simulink model "BLDCspeedcontrollerForGeneralLC"  (R2018b)
settings: Solver=ode15s  StartTime=0  StopTime=10  MaxStep=0.0001  MinStep=1e-9  RelTol=1e-6  AbsTol=1e-9
values from neighbouring files (symbols this model uses):
  battery =     [battery.mat]
  brake =     [brake.mat]
  PE =     [PE.mat]
  pmsm =     [bldc.mat]
undefined symbols (not defined in the file or in its folder): Controller, mech, sigbuilder_block
libraries: simulink x3, simulink_extras x1
settings Model: SimulationMode=accelerator  Creator=dimitriosvogiatzis  LastModifiedBy=dimitriosvogiatzis
settings SolverCC: AutoScaleAbsTol=off  InitialStep=1e-8  MaxConsecutiveZCs=100  MaxConsecutiveMinStep=100  ZeroCrossAlgorithm=Adaptive  AlgebraicLoopSolver=LineSearch
settings DebuggingCC: IgnoredZcDiagnostic=none
settings CodeAppCC: StateflowObjectComments=on

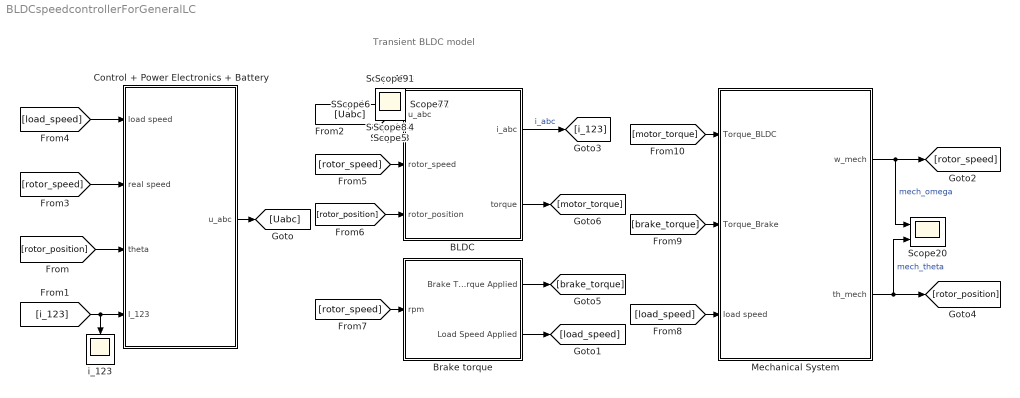
== system BLDCspeedcontrollerForGeneralLC ==
  note: Transient BLDC model
  BLDC : Subsystem
  Brake torque : Subsystem
  Control + Power Electronics + Battery : Subsystem
  Mechanical System : Subsystem
  Scope20 : Scope  NumInputPorts=2
  i_123 : Scope
  Scope{,1..19,21..47} (47 alike) : Scope
  wires:
  BLDC/1(i_abc) -> [i_123]  "i_abc"
  Mechanical System/1(w_mech) -> Scope20/1, [rotor_speed]  "mech_omega"
  Brake torque/1(Brake Torque Applied) -> [brake_torque]
  Mechanical System/2(th_mech) -> Scope20/2, [rotor_position]  "mech_theta"
  [load_speed] -> Control + Power Electronics + Battery/1(load speed)
  [rotor_speed] -> Control + Power Electronics + Battery/2(real speed)
  [rotor_position] -> Control + Power Electronics + Battery/3(theta)
  [i_123] -> Control + Power Electronics + Battery/4(I_123), i_123/1
  [rotor_speed] -> BLDC/2(rotor_speed)
  BLDC/2(torque) -> [motor_torque]
  [rotor_position] -> BLDC/3(rotor_position)
  [rotor_speed] -> Brake torque/1(rpm)
  Brake torque/2(Load Speed Applied) -> [load_speed]
  Control + Power Electronics + Battery/1(u_abc) -> [Uabc]
  [Uabc] -> BLDC/1(u_abc)
  [load_speed] -> Mechanical System/3(load speed)
  [brake_torque] -> Mechanical System/2(Torque_Brake)
  [motor_torque] -> Mechanical System/1(Torque_BLDC)

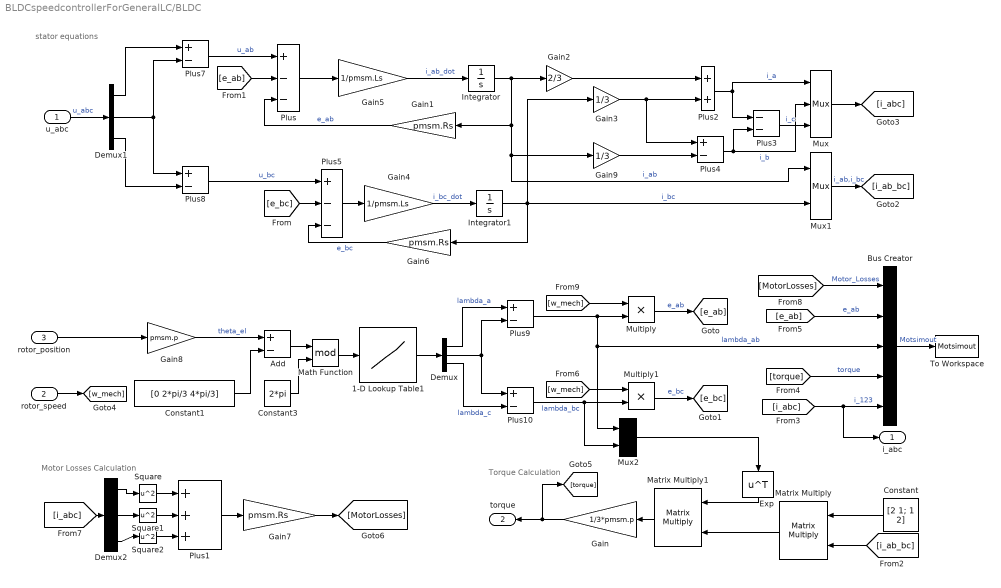
== system BLDCspeedcontrollerForGeneralLC/BLDC ==
  note: Motor Losses Calculation
  note: stator equations
  note: Torque Calculation
  u_abc : Inport
  rotor_speed : Inport  Port=2
  rotor_position : Inport  Port=3
  1-D Lookup Table1 : Lookup_n-D  NumberOfTableDimensions=1  BreakpointsForDimension1=pmsm.phi_tab  Table=pmsm.dlambda_tab  InternalRulePriority=Speed  RndMeth=Simplest  InputSameDT=on
  Add : Sum  Inputs=+-
  Bus Creator : BusCreator  Inputs=5
  Constant : Constant  Value=[2 1; 1 2]
  Constant1 : Constant  Value=[0 2*pi/3 4*pi/3]
  Constant3 : Constant  Value=2*pi
  Demux : Demux  Outputs=3
  Demux1 : Demux  Outputs=3
  Demux2 : Demux  Outputs=3
  Exp : Math  Operator=transpose  OutputSignalType=real  SaturateOnIntegerOverflow=on
  Gain : Gain  Gain=1/3*pmsm.p
  Gain1 : Gain  Gain=pmsm.Rs
  Gain2 : Gain  Gain=2/3
  Gain3 : Gain  Gain=1/3
  Gain4 : Gain  Gain=1/pmsm.Ls
  Gain5 : Gain  Gain=1/pmsm.Ls
  Gain6 : Gain  Gain=pmsm.Rs
  Gain7 : Gain  Gain=pmsm.Rs
  Gain8 : Gain  Gain=pmsm.p
  Gain9 : Gain  Gain=1/3
  Integrator : Integrator
  Integrator1 : Integrator
  Math Function : Math  Operator=mod  SaturateOnIntegerOverflow=on
  Matrix Multiply : Product  Multiplication=Matrix(*)
  Matrix Multiply1 : Product  Multiplication=Matrix(*)
  Multiply : Product
  Multiply1 : Product
  Mux : Mux  Inputs=3
  Mux1 : Mux  Inputs=2
  Mux2 : Mux  Inputs=2
  Plus : Sum  Inputs=+--
  Plus1 : Sum  Inputs=+++
  Plus{4,7..10} (5 alike) : Sum  Inputs=+-
  Plus2 : Sum
  Plus3 : Sum  Inputs=--
  Plus5 : Sum  Inputs=+--
  Square : Math  Operator=square  SaturateOnIntegerOverflow=on
  Square1 : Math  Operator=square  SaturateOnIntegerOverflow=on
  Square2 : Math  Operator=square  SaturateOnIntegerOverflow=on
  To Workspace : ToWorkspace  VariableName=Motsimout  SaveFormat=Timeseries  SampleTime=-1
  i_abc : Outport
  torque : Outport  Port=2
  wires:
  Multiply/1 -> [e_ab]  "e_ab"
  Matrix Multiply/1 -> Matrix Multiply1/2
  Mux2/1 -> Exp/1
  Demux/2 -> Plus9/2, Plus10/1
  Plus10/1 -> Multiply1/2, Mux2/2  "lambda_bc"
  Constant/1 -> Matrix Multiply/1
  [e_bc] -> Plus5/2
  Gain6/1 -> Plus5/3  "e_bc"
  Plus4/1 -> Mux/2, Plus3/2  "i_b"
  1-D Lookup Table1/1 -> Demux/1
  [i_ab_bc] -> Matrix Multiply/2
  Matrix Multiply1/1 -> Gain/1
  Mux1/1 -> [i_ab_bc]  "i_ab,i_bc"
  [e_ab] -> Plus/2
  [i_abc] -> i_abc/1, Bus Creator/5  "i_123"
  Add/1 -> Math Function/1
  Exp/1 -> Matrix Multiply1/1
  Demux/3 -> Plus10/2  "lambda_c"
  [w_mech] -> Multiply/1
  Constant1/1 -> Add/2
  Demux/1 -> Plus9/1  "lambda_a"
  Gain8/1 -> Add/1  "theta_el"
  Math Function/1 -> 1-D Lookup Table1/1
  Gain3/1 -> Plus4/1, Plus2/2
  Plus2/1 -> Mux/1, Plus3/1  "i_a"
  Gain9/1 -> Plus4/2
  Integrator/1 -> Mux1/1, Gain9/1, Gain1/1, Gain2/1  "i_ab"
  Gain1/1 -> Plus/3  "e_ab"
  Gain2/1 -> Plus2/1
  Gain5/1 -> Integrator/1  "i_ab_dot"
  rotor_speed/1 -> [w_mech]
  Gain4/1 -> Integrator1/1  "i_bc_dot"
  Multiply1/1 -> [e_bc]  "e_bc"
  [w_mech] -> Multiply1/1
  Integrator1/1 -> Gain6/1, Mux1/2, Gain3/1  "i_bc"
  Plus/1 -> Gain5/1
  Mux/1 -> [i_abc]
  Plus9/1 -> Mux2/1, Bus Creator/3, Multiply/2  "lambda_ab"
  Plus5/1 -> Gain4/1
  Constant3/1 -> Math Function/2
  Demux1/3 -> Plus8/2
  Demux1/1 -> Plus7/1
  Plus8/1 -> Plus5/1  "u_bc"
  Demux1/2 -> Plus8/1, Plus7/2
  Plus7/1 -> Plus/1  "u_ab"
  u_abc/1 -> Demux1/1  "u_abc"
  rotor_position/1 -> Gain8/1
  Bus Creator/1 -> To Workspace/1  "Motsimout"
  Plus3/1 -> Mux/3  "i_c"
  Gain/1 -> [torque], torque/1
  [torque] -> Bus Creator/4  "torque"
  [e_ab] -> Bus Creator/2  "e_ab"
  [i_abc] -> Demux2/1
  Demux2/1 -> Square/1
  Plus1/1 -> Gain7/1
  Gain7/1 -> [MotorLosses]
  [MotorLosses] -> Bus Creator/1  "Motor_Losses"
  Square/1 -> Plus1/1
  Demux2/2 -> Square1/1
  Square1/1 -> Plus1/2
  Square2/1 -> Plus1/3
  Demux2/3 -> Square2/1

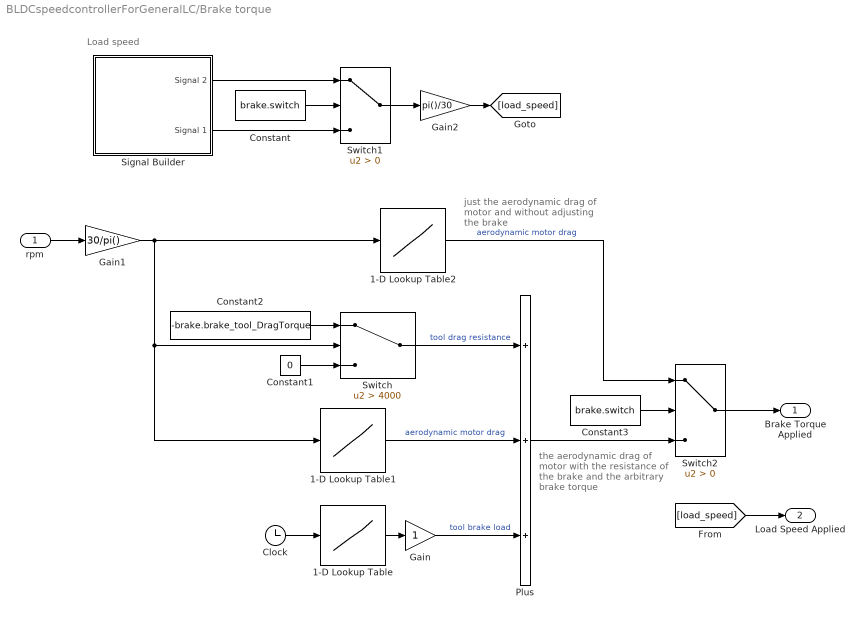
== system BLDCspeedcontrollerForGeneralLC/Brake torque ==
  note: the aerodynamic drag of motor with the resistance of the brake and the arbitrary brake torque
  note: just the aerodynamic drag of motor and without adjusting the brake
  note: Load speed
  rpm : Inport
  1-D Lookup Table : Lookup_n-D  NumberOfTableDimensions=1  BreakpointsForDimension1=brake.brake_time_small  Table=-brake.brake_torque_small  InternalRulePriority=Speed  RndMeth=Simplest  InputSameDT=on
  1-D Lookup Table1 : Lookup_n-D  NumberOfTableDimensions=1  BreakpointsForDimension1=[0,5000,7000,9000,10000,11500,12000]  Table=-1.6*[0,0.28,0.37,0.45,0.5,0.58,0.68]  InternalRulePriority=Speed  RndMeth=Simplest  InputSameDT=on
  1-D Lookup Table2 : Lookup_n-D  NumberOfTableDimensions=1  BreakpointsForDimension1=[0,5000,7000,9000,10000,11500,13000]  Table=-1.6*[0,0.28,0.37,0.45,0.5,0.58,0.68]  InternalRulePriority=Speed  RndMeth=Simplest  InputSameDT=on
  Clock : Clock
  Constant : Constant  Value=brake.switch
  Constant1 : Constant  Value=0
  Constant2 : Constant  Value=-brake.brake_tool_DragTorque
  Constant3 : Constant  Value=brake.switch
  Gain : Gain
  Gain1 : Gain  Gain=30/pi()
  Gain2 : Gain  Gain=pi()/30
  Plus : Sum  Inputs=+++
  Signal Builder : Subsystem  Tag=STV Subsys  LoadFcn=sigbuilder_block('load');  StartFcn=sigbuilder_block('start');  StopFcn=sigbuilder_block('stop');  ClipboardFcn=sigbuilder_block('clipboard');  mask(Sigbuilder block){tuvar=[0:10]}
      mask help: Simulink:masks:SigbuilderBlock_MD
      mask init:
      | if ~strcmp(get_param(bdroot(gcbh),'SimulationStatus'),'stopped') tuvar = sigbuilder_block('maskInit'); end
      settings: CopyFcn=sigbuilder_block('copy');  DeleteFcn=sigbuilder_block('delete');  ModelCloseFcn=sigbuilder_block('modelClose');  PreSaveFcn=sigbuilder_block('preSave');  PauseFcn=sigbuilder_block('pause');  ContinueFcn=sigbuilder_block('continue');  NameChangeFcn=sigbuilder_block('namechange');  OpenFcn=sigbuilder_block('open',[6 30 1428 681.75 ]);  CloseFcn=sigbuilder_block('close');
      mask Display: plot(0, 0, 100, 100,[2, 2, 32, 32, 2], [68, 8, 8, 68, 68],[32, 2], [38, 38], [32, 19, 2],[53, 60, 44], [32, 17, 17, 2],[16, 16, 31, 31]);txt = getActiveGroup(gcbh);text(2, 100, txt,'verticalAlignment', 'top');
  Switch : Switch  Criteria=u2 > Threshold  Threshold=4000
  Switch1 : Switch  Criteria=u2 > Threshold
  Switch2 : Switch  Criteria=u2 > Threshold
  Brake Torque Applied : Outport
  Load Speed Applied : Outport  Port=2
  wires:
  1-D Lookup Table/1 -> Gain/1
  1-D Lookup Table2/1 -> Switch2/1  "aerodynamic motor drag"
  Gain/1 -> Plus/3  "tool brake load"
  Switch2/1 -> Brake Torque Applied/1
  Clock/1 -> 1-D Lookup Table/1
  Plus/1 -> Switch2/3
  1-D Lookup Table1/1 -> Plus/2  "aerodynamic motor drag"
  rpm/1 -> Gain1/1
  Gain1/1 -> 1-D Lookup Table2/1, 1-D Lookup Table1/1, Switch/2
  Constant1/1 -> Switch/3
  Constant2/1 -> Switch/1
  Switch/1 -> Plus/1  "tool drag resistance"
  Signal Builder/2(Signal 1) -> Switch1/3
  Gain2/1 -> [load_speed]
  Switch1/1 -> Gain2/1
  Signal Builder/1(Signal 2) -> Switch1/1
  [load_speed] -> Load Speed Applied/1
  Constant/1 -> Switch1/2
  Constant3/1 -> Switch2/2

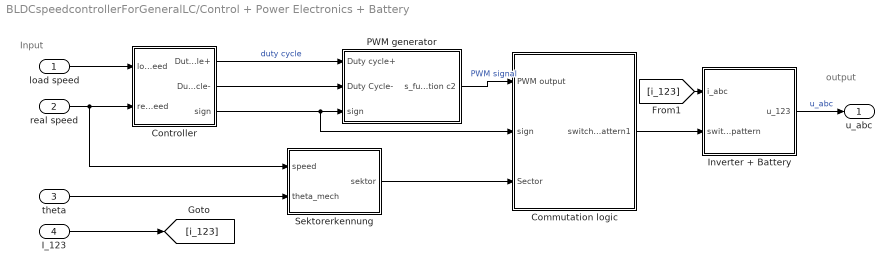
== system BLDCspeedcontrollerForGeneralLC/Control + Power Electronics + Battery ==
  note: output
  note: Input
  load speed : Inport
  real speed : Inport  Port=2
  theta : Inport  Port=3
  I_123 : Inport  Port=4
  Commutation logic : Subsystem
  Controller : Subsystem
  Inverter + Battery : Subsystem
  PWM generator : Subsystem
  Sektorerkennung : Subsystem
  u_abc : Outport
  wires:
  load speed/1 -> Controller/1(load speed)
  theta/1 -> Sektorerkennung/2(theta_mech)
  [i_123] -> Inverter + Battery/1(i_abc)
  Sektorerkennung/1(sektor) -> Commutation logic/3(Sector)
  Controller/1(Duty Cycle+) -> PWM generator/1(Duty cycle+)  "duty cycle"
  Commutation logic/1(switching pattern1) -> Inverter + Battery/2(switching pattern)
  Inverter + Battery/1(u_123) -> u_abc/1  "u_abc"
  real speed/1 -> Sektorerkennung/1(speed), Controller/2(real speed)
  Controller/3(sign) -> Commutation logic/2(sign), PWM generator/3(sign)
  PWM generator/1(s_function c2) -> Commutation logic/1(PWM output)  "PWM signal"
  Controller/2(Duty Cycle-) -> PWM generator/2(Duty Cycle-)
  I_123/1 -> [i_123]

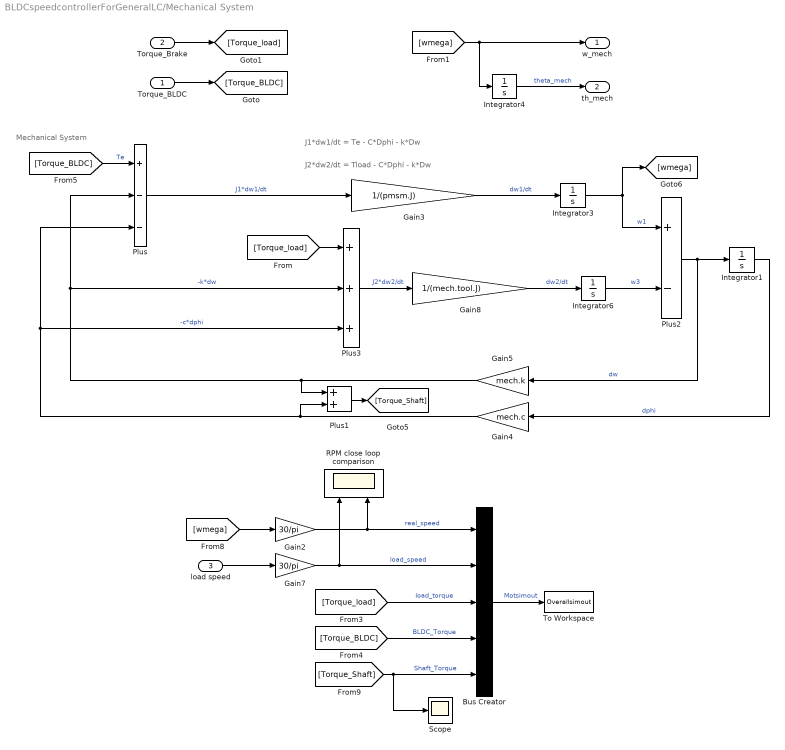
== system BLDCspeedcontrollerForGeneralLC/Mechanical System ==
  note: Mechanical System
  note: J1*dw1/dt = Te - C*Dphi - k*Dw
  note: J2*dw2/dt = Tload - C*Dphi - k*Dw
  Torque_BLDC : Inport
  Torque_Brake : Inport  Port=2
  load speed : Inport  Port=3
  Bus Creator : BusCreator  Inputs=5
  Gain2 : Gain  Gain=30/pi
  Gain3 : Gain  Gain=1/(pmsm.J)
  Gain4 : Gain  Gain=mech.c
  Gain5 : Gain  Gain=mech.k
  Gain7 : Gain  Gain=30/pi
  Gain8 : Gain  Gain=1/(mech.tool.J)
  Integrator{1,3..4,6} (4 alike) : Integrator
  Plus : Sum  Inputs=+--
  Plus1 : Sum
  Plus2 : Sum  Inputs=+-
  Plus3 : Sum  Inputs=+++
  RPM close loop comparison : Scope  NumInputPorts=2
  Scope : Scope
  To Workspace : ToWorkspace  VariableName=Overallsimout  SaveFormat=Timeseries  SampleTime=-1
  w_mech : Outport
  th_mech : Outport  Port=2
  wires:
  Torque_Brake/1 -> [Torque_load]
  Torque_BLDC/1 -> [Torque_BLDC]
  Integrator4/1 -> th_mech/1  "theta_mech"
  Gain4/1 -> Plus1/2, Plus3/3, Plus/3  "-c*dphi"
  Integrator1/1 -> Gain4/1  "dphi"
  Plus1/1 -> [Torque_Shaft]
  Plus2/1 -> Integrator1/1, Gain5/1  "dw"
  Gain3/1 -> Integrator3/1  "dw1/dt"
  Plus/1 -> Gain3/1  "J1*dw1/dt"
  [Torque_BLDC] -> Plus/1  "Te"
  Integrator3/1 -> [wmega], Plus2/1  "w1"
  Gain5/1 -> Plus1/1, Plus3/2, Plus/2  "-k*dw"
  Gain7/1 -> RPM close loop comparison/1, Bus Creator/2  "load_speed"
  Bus Creator/1 -> To Workspace/1  "Motsimout"
  [Torque_load] -> Bus Creator/3  "load_torque"
  [wmega] -> Gain2/1
  load speed/1 -> Gain7/1
  Gain2/1 -> RPM close loop comparison/2, Bus Creator/1  "real_speed"
  [Torque_BLDC] -> Bus Creator/4  "BLDC_Torque"
  [Torque_Shaft] -> Scope/1, Bus Creator/5  "Shaft_Torque"
  [Torque_load] -> Plus3/1
  Plus3/1 -> Gain8/1  "J2*dw2/dt"
  Gain8/1 -> Integrator6/1  "dw2/dt"
  Integrator6/1 -> Plus2/2  "w3"
  [wmega] -> w_mech/1, Integrator4/1

== system BLDCspeedcontrollerForGeneralLC/Brake torque/Signal Builder ==
  Demux : Demux  Tag=STV Demux  Outputs=2
  FromWs : FromWorkspace  Tag=STV FromWs  VariableName=tuvar  SampleTime=0
      SigBuilderData=|
      | common.afterFinalStr = 'Extrapolate'
      | common.sampleTime = 0
      | dataSet.timeRange = [0 10]
      | dataSet.name = 'Group 1'
      | sbobj.Groups.Name = 'Group 1'
      | sbobj.Groups.Signals(1).Name = 'Signal 2'
      | sbobj.Groups.Signals(1).XData = [0 10]
      | sbobj.Groups.Signals(1).YData = [0 200000]
      | sbobj.Groups.Signals(2).Name = 'Signal 1'
      | sbobj.Groups.Signals(2).XData = [0 1.5 3 3.5 5 5.5 8 9 10]
      | sbobj.Groups.Signals(2).YData = [0 4000 4000 6000 6000 8000 8050 10000 0]
  Signal 2 : Outport  Tag=STV Outport
  Signal 1 : Outport  Tag=STV Outport  Port=2
  wires:
  FromWs/1 -> Demux/1
  Demux/1 -> Signal 2/1
  Demux/2 -> Signal 1/1

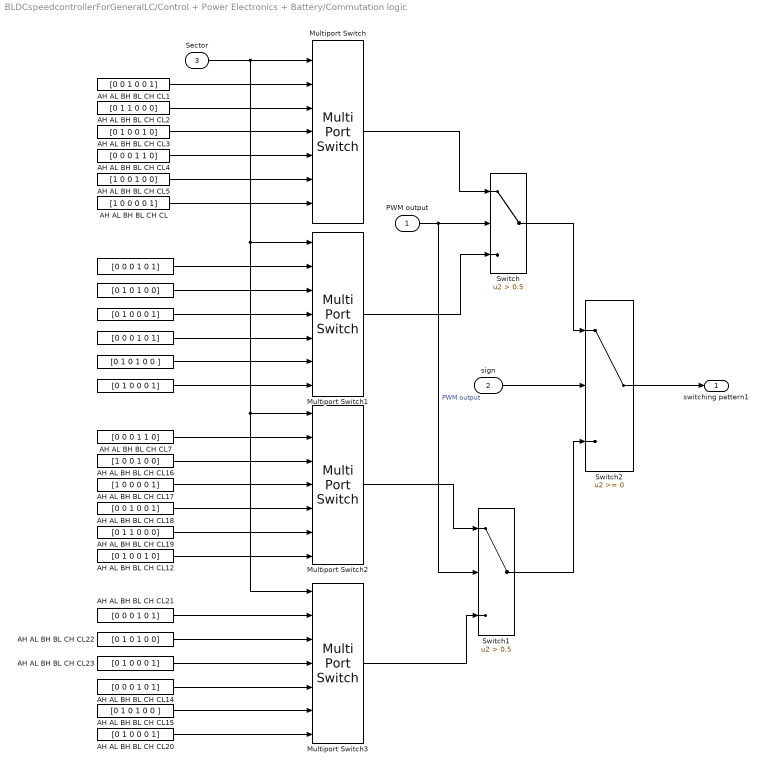
== system BLDCspeedcontrollerForGeneralLC/Control + Power Electronics + Battery/Commutation logic ==
  PWM output : Inport
  sign : Inport  Port=2
  Sector : Inport  Port=3
  " " : Constant  Value=[0 1 0 1 0 0 ]
  "  " : Constant  Value=[0 0 0 1 0 1]
  "   " : Constant  Value=[0 1 0 0 0 1]
  "     " : Constant  Value=[0 1 0 0 0 1]
  "           " : Constant  Value=[0 0 0 1 0 1]
  "                        " : Constant  Value=[0 1 0 1 0 0]
  AH AL BH BL CH CL : Constant  Value=[1 0 0 0 0 1]
  AH AL BH BL CH CL1 : Constant  Value=[0 0 1 0 0 1]
  AH AL BH BL CH CL12 : Constant  Value=[0 1 0 0 1 0]
  AH AL BH BL CH CL14 : Constant  Value=[0 0 0 1 0 1]
  AH AL BH BL CH CL15 : Constant  Value=[0 1 0 1 0 0 ]
  AH AL BH BL CH CL16 : Constant  Value=[1 0 0 1 0 0]
  AH AL BH BL CH CL17 : Constant  Value=[1 0 0 0 0 1]
  AH AL BH BL CH CL18 : Constant  Value=[0 0 1 0 0 1]
  AH AL BH BL CH CL19 : Constant  Value=[0 1 1 0 0 0]
  AH AL BH BL CH CL2 : Constant  Value=[0 1 1 0 0 0]
  AH AL BH BL CH CL20 : Constant  Value=[0 1 0 0 0 1]
  AH AL BH BL CH CL21 : Constant  Value=[0 0 0 1 0 1]
  AH AL BH BL CH CL22 : Constant  Value=[0 1 0 1 0 0]
  AH AL BH BL CH CL23 : Constant  Value=[0 1 0 0 0 1]
  AH AL BH BL CH CL3 : Constant  Value=[0 1 0 0 1 0]
  AH AL BH BL CH CL4 : Constant  Value=[0 0 0 1 1 0]
  AH AL BH BL CH CL5 : Constant  Value=[1 0 0 1 0 0]
  AH AL BH BL CH CL7 : Constant  Value=[0 0 0 1 1 0]
  Multiport Switch{,1..3} (4 alike) : MultiPortSwitch  Inputs=6
  Switch : Switch  Criteria=u2 > Threshold  Threshold=0.5
  Switch1 : Switch  Criteria=u2 > Threshold  Threshold=0.5
  Switch2 : Switch
  switching pattern1 : Outport
  wires:
  Multiport Switch/1 -> Switch/1
  Multiport Switch1/1 -> Switch/3
  PWM output/1 -> Switch1/2, Switch/2  "PWM output"
  Switch/1 -> Switch2/1
  AH AL BH BL CH CL5/1 -> Multiport Switch/6
  AH AL BH BL CH CL4/1 -> Multiport Switch/5
  AH AL BH BL CH CL3/1 -> Multiport Switch/4
  AH AL BH BL CH CL2/1 -> Multiport Switch/3
  AH AL BH BL CH CL1/1 -> Multiport Switch/2
  AH AL BH BL CH CL/1 -> Multiport Switch/7
  "           "/1 -> Multiport Switch1/2
  "                        "/1 -> Multiport Switch1/3
  "     "/1 -> Multiport Switch1/4
  "  "/1 -> Multiport Switch1/5
  " "/1 -> Multiport Switch1/6
  "   "/1 -> Multiport Switch1/7
  AH AL BH BL CH CL20/1 -> Multiport Switch3/7
  AH AL BH BL CH CL15/1 -> Multiport Switch3/6
  AH AL BH BL CH CL14/1 -> Multiport Switch3/5
  AH AL BH BL CH CL23/1 -> Multiport Switch3/4
  AH AL BH BL CH CL22/1 -> Multiport Switch3/3
  AH AL BH BL CH CL21/1 -> Multiport Switch3/2
  AH AL BH BL CH CL12/1 -> Multiport Switch2/7
  AH AL BH BL CH CL7/1 -> Multiport Switch2/2
  AH AL BH BL CH CL16/1 -> Multiport Switch2/3
  AH AL BH BL CH CL17/1 -> Multiport Switch2/4
  AH AL BH BL CH CL18/1 -> Multiport Switch2/5
  AH AL BH BL CH CL19/1 -> Multiport Switch2/6
  Switch1/1 -> Switch2/3
  Sector/1 -> Multiport Switch3/1, Multiport Switch2/1, Multiport Switch1/1, Multiport Switch/1
  Multiport Switch3/1 -> Switch1/3
  Multiport Switch2/1 -> Switch1/1
  sign/1 -> Switch2/2
  Switch2/1 -> switching pattern1/1

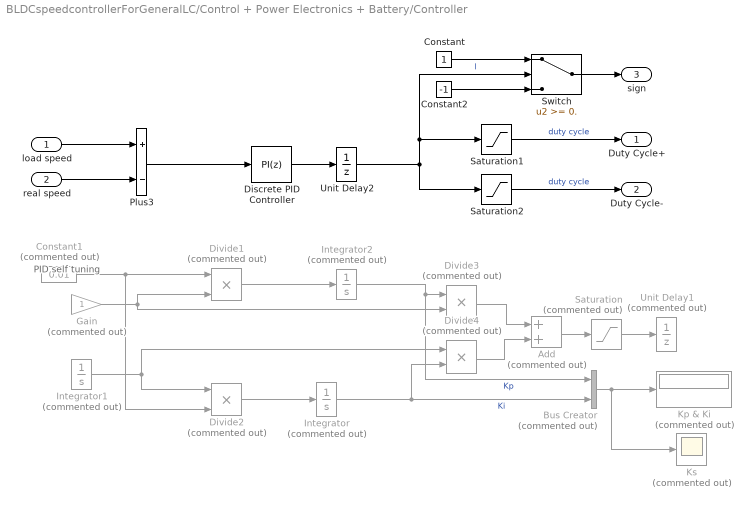
== system BLDCspeedcontrollerForGeneralLC/Control + Power Electronics + Battery/Controller ==
  note: PID self tuning
  load speed : Inport
  real speed : Inport  Port=2
  Add : Sum  Commented=on
  Bus Creator : BusCreator  Commented=on  Inputs=2
  Constant : Constant
  Constant1 : Constant  Commented=on  Value=0.01
  Constant2 : Constant  Value=-1
  Discrete PID Controller : simulink/Continuous/PID Controller  Controller=PI  Form=Parallel  TimeDomain=Discrete-time  SampleTime=-1  IntegratorMethod=Forward Euler  FilterMethod=Forward Euler  ControllerParametersSource=internal  P=PE.controller.kp  I=PE.controller.ki  D=Controller.kd  UseFilter=on  N=100  TunerSelectOption=Transfer Function Based (PID Tuner App)  InitialConditionSource=internal  InitialConditionForIntegrator=0  InitialConditionForFilter=0  DifferentiatorICPrevScaledInput=0  ExternalReset=none  TrackingMode=off  Kt=1  LimitOutput=off  UpperSaturationLimit=2  LowerSaturationLimit=-1  LinearizeAsGain=off  AntiWindupMode=none  Kb=1  POutMin=[]  POutMax=[]  IOutMin=[]  IOutMax=[]  DOutMin=[]  DOutMax=[]  NOutMin=[]  NOutMax=[]  SumOutMin=[]  SumOutMax=[]  SaturationOutMin=[]  SaturationOutMax=[]  PParamMin=[]  PParamMax=[]  IParamMin=[]  IParamMax=[]  DParamMin=[]  DParamMax=[]  NParamMin=[]  NParamMax=[]  KbParamMin=[]  KbParamMax=[]  KtParamMin=[]  KtParamMax=[]  KbOutMin=[]  KbOutMax=[]  KtOutMin=[]  KtOutMax=[]  IntegratorOutMin=[]  IntegratorOutMax=[]  FilterOutMin=[]  FilterOutMax=[]  SumI1OutMin=[]  SumI1OutMax=[]  SumI2OutMin=[]  SumI2OutMax=[]  SumI3OutMin=[]  SumI3OutMax=[]  SumI4OutMin=[]  SumI4OutMax=[]  SumDOutMin=[]  SumDOutMax=[]  DifferentiatorOutMin=[]  DifferentiatorOutMax=[]  FilterDiffOutCoefMin=[]  FilterDiffOutCoefMax=[]  ReciprocalOutMin=[]  ReciprocalOutMax=[]  SumDenOutMin=[]  SumDenOutMax=[]  SumNumOutMin=[]  SumNumOutMax=[]  DivideOutMin=[]  DivideOutMax=[]  IntegratorContinuousStateAttributes=''  IntegratorStateMustResolveToSignalObject=off  IntegratorRTWStateStorageClass=Auto  FilterContinuousStateAttributes=''  FilterStateMustResolveToSignalObject=off  FilterRTWStateStorageClass=Auto  ParallelPVariant=InternalParameters  IdealPVariant=Disabled  IVariant=InternalParameters  DVariant=Disabled  IntegratorVariant=Discrete  SatVariant=Disabled  AWVariant=Passthrough  PCopyVariant=Disabled  TRVariant=Disabled  FdbkBlocksVariant=Forward  IdealPFdbkVariant=Disabled  SatFdbkVariant=Disabled  DerivativeFilterVariant=Disabled  NVariant=Disabled  NCopyVariant=Disabled_SignalSpec  FilterICVariant=Disabled  IntegratorICVariant=InternalICs  ExternalResetVariant=Disabled  TRSumVariant=Passthrough  SumFdbkVariant=Disabled  SumVariant=Sum_PI
  Divide1 : Product  Commented=on  Inputs=***
  Divide2 : Product  Commented=on  Inputs=***
  Divide3 : Product  Commented=on  Inputs=**
  Divide4 : Product  Commented=on  Inputs=**
  Gain : Gain  Commented=on
  Integrator : Integrator  Commented=on  ZeroCross=off
  Integrator1 : Integrator  Commented=on  InitialCondition=-2  ZeroCross=off
  Integrator2 : Integrator  Commented=on  ZeroCross=off
  "Kp & Ki " : Display  Commented=on
  Ks : Scope  Commented=on
  Plus3 : Sum  Inputs=+-
  Saturation : Saturate  Commented=on  UpperLimit=1000  LowerLimit=-1000
  Saturation1 : Saturate  UpperLimit=1  LowerLimit=0
  Saturation2 : Saturate  UpperLimit=0  LowerLimit=-1
  Switch : Switch  Threshold=0.
  Unit Delay1 : UnitDelay  Commented=on  SampleTime=-1
  Unit Delay2 : UnitDelay  SampleTime=-1
  Duty Cycle+ : Outport
  Duty Cycle- : Outport  Port=2
  sign : Outport  Port=3
  wires:
  Saturation/1 -> Unit Delay1/1
  Bus Creator/1 -> Ks/1, "Kp & Ki "/1
  Integrator2/1 -> Bus Creator/1, Divide3/1  "Kp"
  Integrator1/1 -> Divide4/1, Divide2/1
  Divide3/1 -> Add/1
  Divide4/1 -> Add/2
  Divide2/1 -> Integrator/1
  Integrator/1 -> Divide4/2, Bus Creator/2  "Ki"
  Add/1 -> Saturation/1
  Divide1/1 -> Integrator2/1
  Gain/1 -> Divide3/2, Divide1/3
  Constant1/1 -> Divide2/3, Divide1/1
  Plus3/1 -> Discrete PID Controller/1
  Discrete PID Controller/1 -> Unit Delay2/1
  Constant/1 -> Switch/1
  Constant2/1 -> Switch/3
  Switch/1 -> sign/1
  Unit Delay2/1 -> Switch/2, Saturation1/1, Saturation2/1  "l"
  Saturation1/1 -> Duty Cycle+/1  "duty cycle"
  Saturation2/1 -> Duty Cycle-/1  "duty cycle"
  load speed/1 -> Plus3/1
  real speed/1 -> Plus3/2

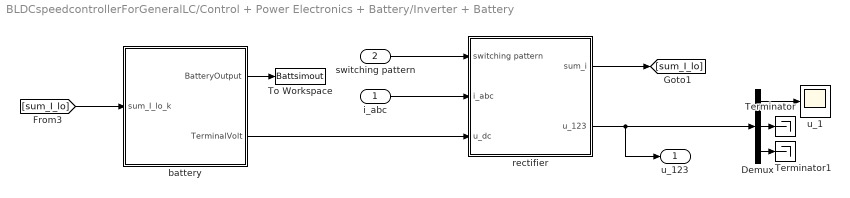
== system BLDCspeedcontrollerForGeneralLC/Control + Power Electronics + Battery/Inverter + Battery ==
  i_abc : Inport
  switching pattern : Inport  Port=2
  Demux : Demux  Outputs=3
  Terminator : Terminator
  Terminator1 : Terminator
  To Workspace : ToWorkspace  VariableName=Battsimout  SaveFormat=Timeseries  SampleTime=-1
  battery : Subsystem
  rectifier : Subsystem
  u_1 : Scope
  u_123 : Outport
  wires:
  [sum_I_lo] -> battery/1(sum_I_lo_k)
  rectifier/2(u_123) -> Demux/1, u_123/1
  battery/2(TerminalVolt) -> rectifier/3(u_dc)
  rectifier/1(sum_i) -> [sum_I_lo]
  Demux/1 -> u_1/1
  Demux/2 -> Terminator/1
  Demux/3 -> Terminator1/1
  switching pattern/1 -> rectifier/1(switching pattern)
  battery/1(BatteryOutput) -> To Workspace/1
  i_abc/1 -> rectifier/2(i_abc)

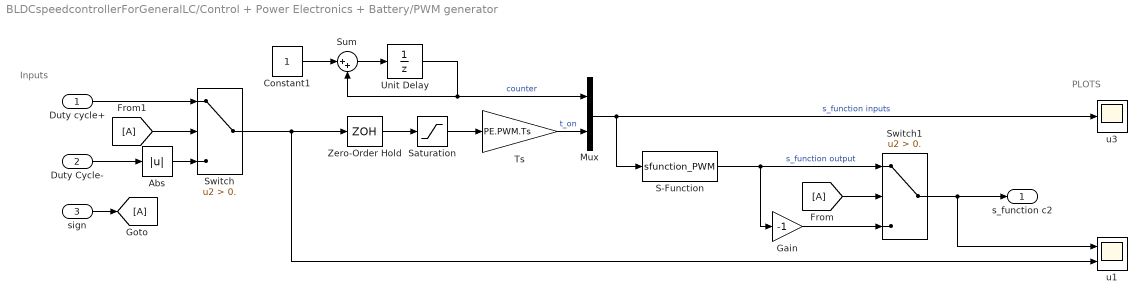
== system BLDCspeedcontrollerForGeneralLC/Control + Power Electronics + Battery/PWM generator ==
  note: Inputs
  note: PLOTS
  Duty cycle+ : Inport
  Duty Cycle- : Inport  Port=2
  sign : Inport  Port=3
  Abs : Abs
  Constant1 : Constant
  Gain : Gain  Gain=-1
  Mux : Mux  Inputs=2
  S-Function : S-Function  FunctionName=sfunction_PWM  Parameters=PE.PWM.Ts  SFunctionDeploymentMode=off  EnableBusSupport=off
  Saturation : Saturate  UpperLimit=1  LowerLimit=0
  Sum : Sum  Inputs=|++
  Switch : Switch  Criteria=u2 > Threshold  Threshold=0.
  Switch1 : Switch  Criteria=u2 > Threshold  Threshold=0.
  Ts : Gain  Gain=PE.PWM.Ts
  Unit Delay : UnitDelay  SampleTime=PE.PWM.Ts
  Zero-Order Hold : ZeroOrderHold  SampleTime=PE.PWM.Ts
  u1 : Scope  NumInputPorts=2
  u3 : Scope
  s_function c2 : Outport
  wires:
  Duty cycle+/1 -> Switch/1
  Constant1/1 -> Sum/1
  S-Function/1 -> Gain/1, Switch1/1  "s_function output"
  Mux/1 -> S-Function/1, u3/1  "s_function inputs"
  Sum/1 -> Unit Delay/1
  Unit Delay/1 -> Sum/2, Mux/1  "counter"
  Ts/1 -> Mux/2  "t_on"
  Saturation/1 -> Ts/1
  Zero-Order Hold/1 -> Saturation/1
  Duty Cycle-/1 -> Abs/1
  sign/1 -> [A]
  Switch/1 -> Zero-Order Hold/1, u1/2
  Abs/1 -> Switch/3
  Gain/1 -> Switch1/3
  Switch1/1 -> u1/1, s_function c2/1
  [A] -> Switch1/2
  [A] -> Switch/2

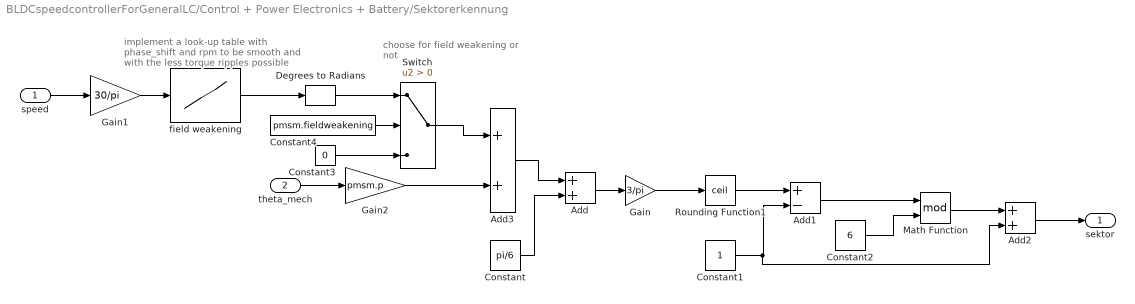
== system BLDCspeedcontrollerForGeneralLC/Control + Power Electronics + Battery/Sektorerkennung ==
  note: choose for field weakening or not
  note: implement a look-up table with phase_shift and rpm to be smooth and with the less torque ripples possible
  speed : Inport
  theta_mech : Inport  Port=2
  Add : Sum
  Add1 : Sum  Inputs=+-
  Add2 : Sum
  Add3 : Sum
  Constant : Constant  Value=pi/6
  Constant1 : Constant
  Constant2 : Constant  Value=6
  Constant3 : Constant  Value=0
  Constant4 : Constant  Value=pmsm.fieldweakening
  Degrees to Radians : simulink_extras/Transformations/Degrees to Radians
  Gain : Gain  Gain=3/pi
  Gain1 : Gain  Gain=30/pi
  Gain2 : Gain  Gain=pmsm.p
  Math Function : Math  Operator=mod  SaturateOnIntegerOverflow=on
  Rounding Function1 : Rounding  Operator=ceil
  Switch : Switch  Criteria=u2 > Threshold
  field weakening : Lookup_n-D  NumberOfTableDimensions=1  BreakpointsForDimension1=pmsm.Speed_phase_shift  Table=pmsm.Phase_shift  InternalRulePriority=Speed  RndMeth=Simplest  InputSameDT=on
  sektor : Outport
  wires:
  Math Function/1 -> Add2/1
  theta_mech/1 -> Gain2/1
  Add1/1 -> Math Function/1
  Add2/1 -> sektor/1
  Rounding Function1/1 -> Add1/1
  Add/1 -> Gain/1
  Constant/1 -> Add/2
  Constant2/1 -> Math Function/2
  Gain/1 -> Rounding Function1/1
  Constant1/1 -> Add2/2, Add1/2
  Gain2/1 -> Add3/2
  Add3/1 -> Add/1
  Gain1/1 -> field weakening/1
  field weakening/1 -> Degrees to Radians/1
  speed/1 -> Gain1/1
  Degrees to Radians/1 -> Switch/1
  Switch/1 -> Add3/1
  Constant3/1 -> Switch/3
  Constant4/1 -> Switch/2

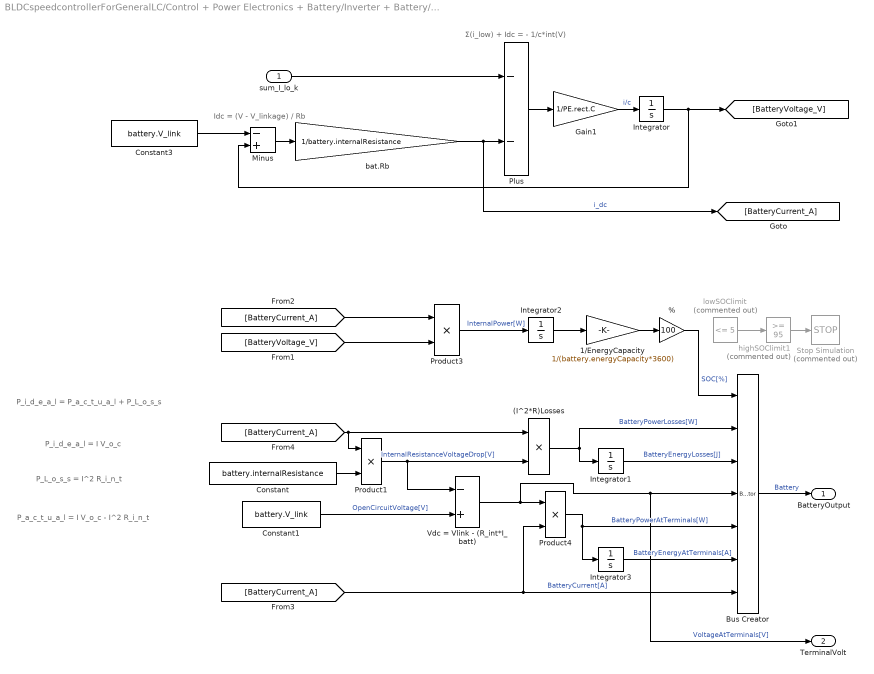
== system BLDCspeedcontrollerForGeneralLC/Control + Power Electronics + Battery/Inverter + Battery/battery ==
  note: Σ(i_low) + Idc = - 1/c*int(V)
  note: Idc = (V - V_linkage) / Rb
  note: P_a_c_t_u_a_l = I V_o_c - I^2 R_i_n_t
  note: P_L_o_s_s = I^2 R_i_n_t
  note: P_i_d_e_a_l = I V_o_c
  note: P_i_d_e_a_l = P_a_c_t_u_a_l + P_L_o_s_s
  sum_I_lo_k : Inport
  % : Gain  Gain=100
  (I^2*R)Losses : Product  RndMeth=Zero
  1/EnergyCapacity : Gain  Gain=1/(battery.energyCapacity*3600)
  Bus Creator : BusCreator  Inputs=7
  Constant : Constant  Value=battery.internalResistance
  Constant1 : Constant  Value=battery.V_link
  Constant3 : Constant  Value=battery.V_link
  Gain1 : Gain  Gain=1/PE.rect.C
  Integrator : Integrator  InitialCondition=battery.V_link
  Integrator1 : Integrator  ZeroCross=off
  Integrator2 : Integrator  InitialCondition=battery.energyCapacity*3600*battery.initialSOC  ZeroCross=off
  Integrator3 : Integrator
  Minus : Sum  Inputs=-+
  Plus : Sum  Inputs=--
  Product1 : Product  RndMeth=Zero
  Product3 : Product  RndMeth=Zero
  Product4 : Product  RndMeth=Zero
  Stop Simulation : Stop  Commented=on
  Vdc = Vlink - (R_int*I_batt) : Sum  Inputs=-+
  "bat.Rb " : Gain  Gain=1/battery.internalResistance
  highSOClimit1 : simulink/Logic and Bit Operations/Compare To Constant  Commented=on  relop=>=  const=95  OutDataTypeStr=boolean
  lowSOClimit : simulink/Logic and Bit Operations/Compare To Constant  Commented=on  relop=<=  const=5  OutDataTypeStr=boolean
  BatteryOutput : Outport
  TerminalVolt : Outport  Port=2
  wires:
  "bat.Rb "/1 -> [BatteryCurrent_A], Plus/2  "i_dc"
  Plus/1 -> Gain1/1
  Constant3/1 -> Minus/1
  sum_I_lo_k/1 -> Plus/1
  Minus/1 -> "bat.Rb "/1
  Integrator/1 -> [BatteryVoltage_V], Minus/2
  Gain1/1 -> Integrator/1  "i/c"
  Integrator2/1 -> 1/EnergyCapacity/1
  Product3/1 -> Integrator2/1  "InternalPower[W]"
  Vdc = Vlink - (R_int*I_batt)/1 -> Product4/1, TerminalVolt/1, Bus Creator/4  "VoltageAtTerminals[V]"
  %/1 -> Bus Creator/1  "SOC[%]"
  highSOClimit1/1 -> Stop Simulation/1
  [BatteryCurrent_A] -> Product1/1, (I^2*R)Losses/1
  Integrator3/1 -> Bus Creator/6  "BatteryEnergyAtTerminals[A]"
  Bus Creator/1 -> BatteryOutput/1  "Battery"
  (I^2*R)Losses/1 -> Integrator1/1, Bus Creator/2  "BatteryPowerLosses[W]"
  Integrator1/1 -> Bus Creator/3  "BatteryEnergyLosses[J]"
  1/EnergyCapacity/1 -> %/1
  Constant/1 -> Product1/2
  Product1/1 -> Vdc = Vlink - (R_int*I_batt)/1, (I^2*R)Losses/2  "InternalResistanceVoltageDrop[V]"
  [BatteryVoltage_V] -> Product3/2
  Product4/1 -> Integrator3/1, Bus Creator/5  "BatteryPowerAtTerminals[W]"
  Constant1/1 -> Vdc = Vlink - (R_int*I_batt)/2  "OpenCircuitVoltage[V]"
  [BatteryCurrent_A] -> Product3/1
  [BatteryCurrent_A] -> Product4/2, Bus Creator/7  "BatteryCurrent[A]"
  lowSOClimit/1 -> highSOClimit1/1

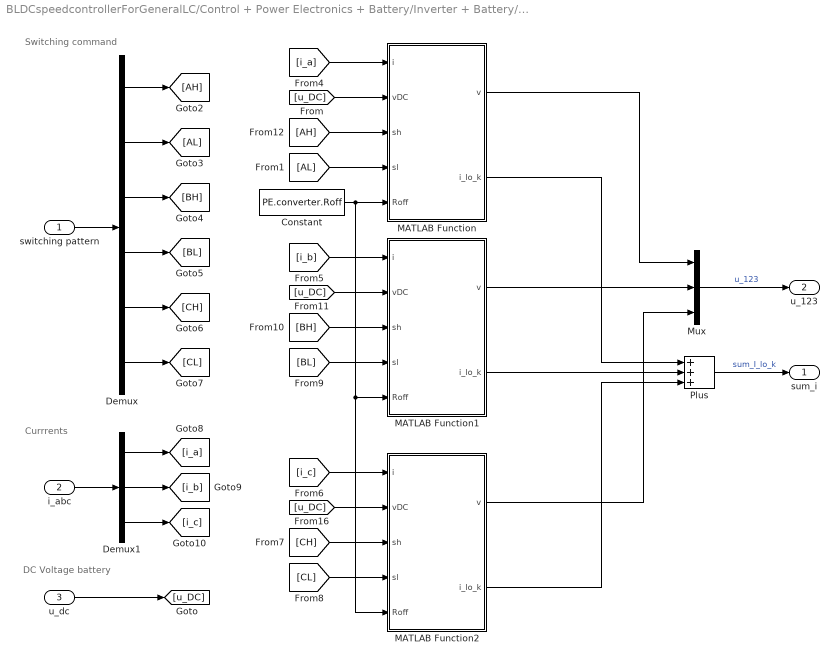
== system BLDCspeedcontrollerForGeneralLC/Control + Power Electronics + Battery/Inverter + Battery/rectifier ==
  note: DC Voltage battery
  note: Currrents
  note: Switching command
  switching pattern : Inport
  i_abc : Inport  Port=2
  u_dc : Inport  Port=3
  Constant : Constant  Value=PE.converter.Roff
  Demux : Demux  Outputs=6
  Demux1 : Demux  Outputs=3
  MATLAB Function : MATLAB Function  TreatAsAtomicUnit=on
  MATLAB Function1 : MATLAB Function  TreatAsAtomicUnit=on
  MATLAB Function2 : MATLAB Function  TreatAsAtomicUnit=on
  Mux : Mux  Inputs=3
  Plus : Sum  Inputs=+++
  sum_i : Outport
  u_123 : Outport  Port=2
  wires:
  [u_DC] -> MATLAB Function/2(vDC)
  switching pattern/1 -> Demux/1
  Mux/1 -> u_123/1  "u_123"
  u_dc/1 -> [u_DC]
  Demux/4 -> [BL]
  Demux/5 -> [CH]
  Demux/2 -> [AL]
  Demux/3 -> [BH]
  Demux/6 -> [CL]
  Demux/1 -> [AH]
  [AH] -> MATLAB Function/3(sh)
  i_abc/1 -> Demux1/1
  Demux1/1 -> [i_a]
  Demux1/2 -> [i_b]
  Demux1/3 -> [i_c]
  [i_a] -> MATLAB Function/1(i)
  [AL] -> MATLAB Function/4(sl)
  [BL] -> MATLAB Function1/4(sl)
  [i_b] -> MATLAB Function1/1(i)
  [BH] -> MATLAB Function1/3(sh)
  [u_DC] -> MATLAB Function1/2(vDC)
  [u_DC] -> MATLAB Function2/2(vDC)
  [CH] -> MATLAB Function2/3(sh)
  [i_c] -> MATLAB Function2/1(i)
  [CL] -> MATLAB Function2/4(sl)
  MATLAB Function/1(v) -> Mux/1
  MATLAB Function1/1(v) -> Mux/2
  MATLAB Function2/1(v) -> Mux/3
  Plus/1 -> sum_i/1  "sum_I_lo_k"
  Constant/1 -> MATLAB Function2/5(Roff), MATLAB Function1/5(Roff), MATLAB Function/5(Roff)
  MATLAB Function1/2(i_lo_k) -> Plus/2
  MATLAB Function/2(i_lo_k) -> Plus/1
  MATLAB Function2/2(i_lo_k) -> Plus/3

== matlab function BLDCspeedcontrollerForGeneralLC/Control + Power Electronics + Battery/Inverter + Battery/rectifier/MATLAB Function ==
  data: i input; v output; vDC input; i_lo_k output; sh input; sl input; Roff input
function [v,i_lo_k] = rectif(i,vDC, sh, sl,Roff)


if (sh == 0 && sl == 1)         % The high switch is open
    v = 0;
    i_lo_k =  -i + vDC/Roff;
elseif (sh == 1 && sl == 0)     % The low switch is open
    v = vDC ;
    i_lo_k =  vDC/Roff;
elseif (sh == 0 && sl == 0)     % Both switch is open
    v = min(max((vDC - i*Roff)/2,0),vDC) ; 
        if i<=0
        i_lo_k = v/Roff;
        else
        i_lo_k = -i+(vDC-v)/Roff;
        end
else     
    v = 0;
    i_lo_k = 0;
end

== matlab function BLDCspeedcontrollerForGeneralLC/Control + Power Electronics + Battery/Inverter + Battery/rectifier/MATLAB Function1 ==
  data: i input; v output; vDC input; i_lo_k output; sh input; sl input; Roff input
function [v,i_lo_k] = rectif(i,vDC, sh, sl,Roff)


if (sh == 0 && sl == 1)         % The high switch is open
    v = 0;
    i_lo_k =  -i + vDC/Roff;
elseif (sh == 1 && sl == 0)     % The low switch is open
    v = vDC ;
    i_lo_k =  vDC/Roff;
elseif (sh == 0 && sl == 0)     % Both switch is open
    v = min(max((vDC - i*Roff)/2,0),vDC) ; 
        if i<=0
        i_lo_k = v/Roff;
        else
        i_lo_k = -i+(vDC-v)/Roff;
        end
else     
    v = 0;
    i_lo_k = 0;
end

== matlab function BLDCspeedcontrollerForGeneralLC/Control + Power Electronics + Battery/Inverter + Battery/rectifier/MATLAB Function2 ==
  data: i input; v output; vDC input; i_lo_k output; sh input; sl input; Roff input
function [v,i_lo_k] = rectif(i,vDC, sh, sl,Roff)


if (sh == 0 && sl == 1)         % The high switch is open
    v = 0;
    i_lo_k =  -i + vDC/Roff;
elseif (sh == 1 && sl == 0)     % The low switch is open
    v = vDC ;
    i_lo_k =  vDC/Roff;
elseif (sh == 0 && sl == 0)     % Both switch is open
    v = min(max((vDC - i*Roff)/2,0),vDC) ; 
        if i<=0
        i_lo_k = v/Roff;
        else
        i_lo_k = -i+(vDC-v)/Roff;
        end
else     
    v = 0;
    i_lo_k = 0;
end
